simulink model "W1Q9"  (R2020a)
settings: Solver=VariableStepAuto  StartTime=0.0  StopTime=10.0  RelTol=1e-3
values from neighbouring files (symbols this model uses):
  B = 0.0001    [para.m]
  J = 0.00002    (= 2e-05)    [para.m]
  Te = 200    [para.m]
  TL = 150    [para.m]
settings Model: Creator=Vinayak  LastModifiedBy=Vinayak

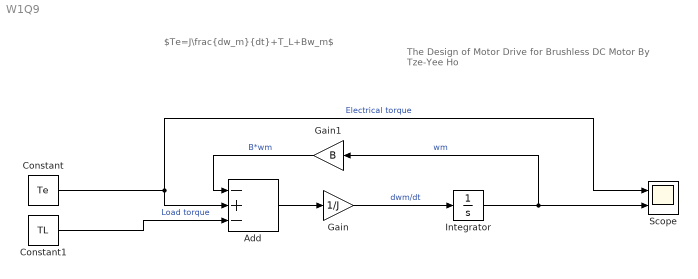
== system W1Q9 ==
  note: The Design of Motor Drive for Brushless DC Motor
      | By Tze-Yee Ho
  note: $Te=J\frac{dw_m}{dt}+T_L+Bw_m$
  Add : Sum  Inputs=-+-
  Constant : Constant  Value=Te
  Constant1 : Constant  Value=TL
  Gain : Gain  Gain=1/J
  Gain1 : Gain  Gain=B
  Integrator : Integrator
  Scope : Scope  NumInputPorts=2
  wires:
  Integrator/1 -> Gain1/1, Scope/2  "wm"
  Add/1 -> Gain/1
  Gain/1 -> Integrator/1  "dwm/dt"
  Constant/1 -> Add/2, Scope/1  "Electrical torque"
  Constant1/1 -> Add/3  "Load torque"
  Gain1/1 -> Add/1  "B*wm"
